simulink model "ControlOptimoInverso"  (R2025a)
settings: Solver=ode8  StartTime=0.0  StopTime=100  FixedStep=1e-3  RelTol=1e-3
libraries: simulink x1, spsRMSLib x1
settings Model: Creator=440G5  LastModifiedBy=440G5

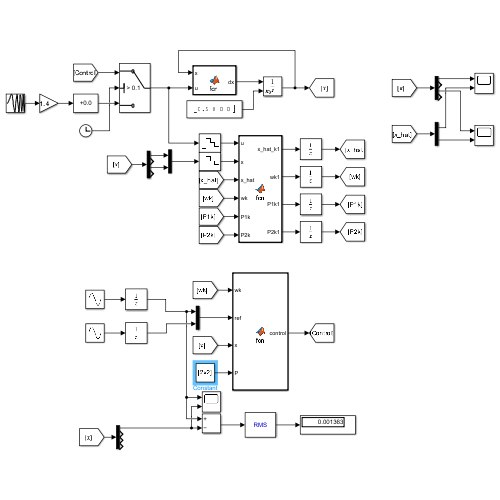
[thumbnail: Simulink's stored preview of the top-level diagram]
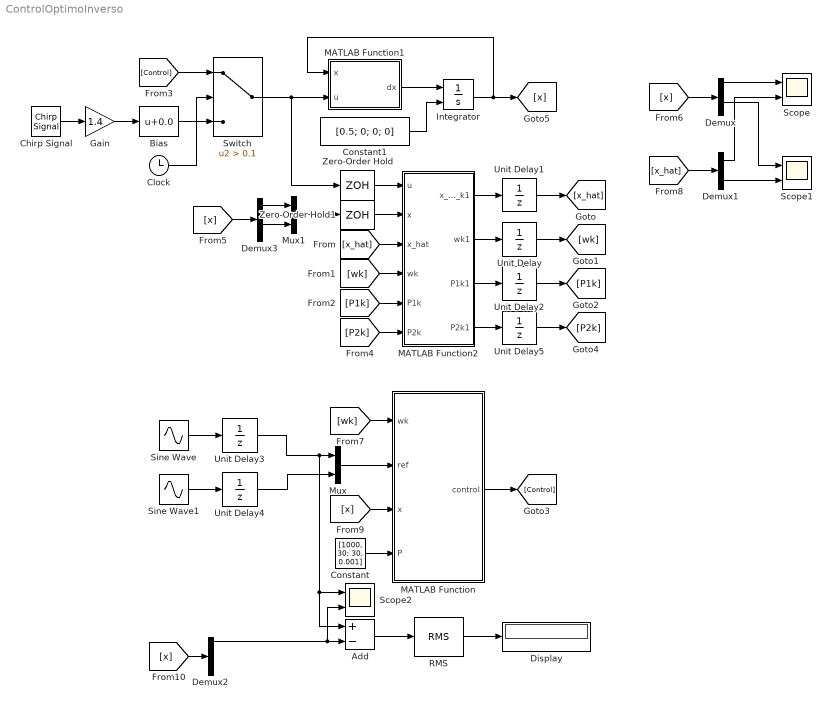
== system ControlOptimoInverso ==
  Add : Sum  Inputs=+-
  Bias : Bias  Bias=0.0  SaturateOnIntegerOverflow=off
  Chirp Signal : simulink/Sources/Chirp Signal  f1=0.08  T=10  f2=1
  Clock : Clock
      settings: Decimation=5
  Constant : Constant  Value=[1000, 30; 30, 0.001]
  Constant1 : Constant  Value=[0.5; 0; 0; 0]
  Demux : Demux
  Demux1 : Demux  Outputs=2
  Demux2 : Demux
  Demux3 : Demux
  Display : Display
  Gain : Gain  Gain=1.4
  Integrator : Integrator  InitialConditionSource=external
  MATLAB Function : MATLAB Function  TreatAsAtomicUnit=on
  MATLAB Function1 : MATLAB Function  TreatAsAtomicUnit=on
  MATLAB Function2 : MATLAB Function  TreatAsAtomicUnit=on
  Mux : Mux  Inputs=2
  Mux1 : Mux  Inputs=2
  RMS : spsRMSLib/RMS  TrueRMS=on  Freq=60  RMSInit=120  Ts=0
  Scope : Scope  NumInputPorts=2
      settings: ActiveDisplayYMinimum=-0.41183517995151714  ActiveDisplayYMaximum=0.922457634321867
  Scope1 : Scope  NumInputPorts=2
      settings: ActiveDisplayYMinimum=-0.72359460835221556  ActiveDisplayYMaximum=1.2933274161774539
  Scope2 : Scope  NumInputPorts=2
      settings: ActiveDisplayYMinimum=-0.92610552404399937  ActiveDisplayYMaximum=0.97588104782378549  DataLoggingVariableName=ScopeData2
  Sine Wave : Sin  Amplitude=0.35  SampleTime=0
  Sine Wave1 : Sin  Amplitude=0.5  SampleTime=0
  Switch : Switch  Criteria=u2 > Threshold  Threshold=0.1  SaturateOnIntegerOverflow=off  InputSameDT=off
  Unit Delay : UnitDelay  InitialCondition=[rand(1,4)]  SampleTime=-1  HasFrameUpgradeWarning=on
  Unit Delay1 : UnitDelay  SampleTime=-1  HasFrameUpgradeWarning=on
  Unit Delay2 : UnitDelay  InitialCondition=eye(2)*5e4  SampleTime=-1  HasFrameUpgradeWarning=on
  Unit Delay3 : UnitDelay  SampleTime=-1  HasFrameUpgradeWarning=on
  Unit Delay4 : UnitDelay  SampleTime=-1  HasFrameUpgradeWarning=on
  Unit Delay5 : UnitDelay  InitialCondition=eye(2)*5e4  SampleTime=-1  HasFrameUpgradeWarning=on
  Zero-Order Hold : ZeroOrderHold  SampleTime=-1
  Zero-Order Hold1 : ZeroOrderHold  SampleTime=-1
  wires:
  Chirp Signal/1 -> Gain/1
  Gain/1 -> Bias/1
  Bias/1 -> Switch/3
  Clock/1 -> Switch/2
  [Control] -> Switch/1
  MATLAB Function/1(control) -> [Control]
  Mux/1 -> MATLAB Function/2(ref)
  Constant/1 -> MATLAB Function/4(P)
  Sine Wave/1 -> Unit Delay3/1
  Sine Wave1/1 -> Unit Delay4/1
  Unit Delay3/1 -> Add/1, Scope2/1, Mux/1
  Unit Delay4/1 -> Mux/2
  [wk] -> MATLAB Function/1(wk)
  Unit Delay1/1 -> [x_hat]
  MATLAB Function2/2(wk1) -> Unit Delay/1
  [x] -> Demux/1
  [P2k] -> MATLAB Function2/6(P2k)
  Demux1/1 -> Scope/2
  [x_hat] -> Demux1/1
  MATLAB Function2/3(P1k1) -> Unit Delay2/1
  [wk] -> MATLAB Function2/4(wk)
  Unit Delay5/1 -> [P2k]
  Constant1/1 -> Integrator/2
  Demux1/2 -> Scope1/2
  Integrator/1 -> [x], MATLAB Function1/1(x)
  MATLAB Function2/1(x_hat_k1) -> Unit Delay1/1
  MATLAB Function1/1(dx) -> Integrator/1
  Zero-Order Hold/1 -> MATLAB Function2/1(u)
  Unit Delay/1 -> [wk]
  Unit Delay2/1 -> [P1k]
  [x_hat] -> MATLAB Function2/3(x_hat)
  Demux/1 -> Scope/1
  MATLAB Function2/4(P2k1) -> Unit Delay5/1
  Zero-Order Hold1/1 -> MATLAB Function2/2(x)
  [P1k] -> MATLAB Function2/5(P1k)
  [x] -> MATLAB Function/3(x)
  [x] -> Demux2/1
  Switch/1 -> Zero-Order Hold/1, MATLAB Function1/2(u)
  Demux3/1 -> Mux1/1
  Mux1/1 -> Zero-Order Hold1/1
  [x] -> Demux3/1
  Demux3/3 -> Mux1/2
  Demux/3 -> Scope1/1
  Demux2/1 -> Scope2/2, Add/2
  Add/1 -> RMS/1
  RMS/1 -> Display/1

== matlab function ControlOptimoInverso/MATLAB Function1 ==
  data: x input; u input; dx output
function dx = fcn(x, u)

m1 = 1;
m2 = 2;
k1 = 2;
k2 = 3;
b1 = 0.2;
b2 = 0.4;

dx1 = x(3);
dx2 = x(4);
dx3 = u/m1 -(k1/m1)*x(1) + (k1/m1)*x(2) -(b1/m1)*x(3) + (b1/m1)*x(4);
dx4 = (k1/m2)*x(1) - (k1/m2)*x(2) + (b1/m2)*x(3) -(b1/m2)*x(4) -(k2/m2)*x(2) -(b2/m2)*x(4);

dx = [dx1; dx2; dx3; dx4];

% function dx  = fcn(x, u)
% g = 9.81;  
% l = 1;     
% m = 1;     
% b = 0.5;   
% 
% x1 = x(1);  
% x2 = x(2);
% 
% dx1 = x2;
% dx2 = (g/l)*sin(x1) - (b/(m*l^2))*x2 + u/(m*l^2);
% 
% dx = [dx1; dx2];
% 
% y = x1;

== matlab function ControlOptimoInverso/MATLAB Function ==
  data: wk input; control output; ref input; x input; P input
function control  = fcn(wk, ref, x, P)

%% Constant weights
w_1 = 0.15;

%% Neural model
f1 = [wk(1)*tanh(x(2)) + wk(2)*tanh(x(1)); wk(3)*tanh(x(1)) + wk(4)*tanh(x(2))];
g1 = [0; w_1];

%% Control law
R = 1;
control = -1/2*(R+1/2*g1'*P*g1)\g1'*P*(f1 -[ref(1); ref(2)]);
end

== matlab function ControlOptimoInverso/MATLAB Function2 ==
  data: u input; x input; x_hat input; wk input; P1k input; P2k input; x_hat_k1 output; wk1 output; P1k1 output; P2k1 output
function [x_hat_k1, wk1, P1k1, P2k1] = fcn(u, x, x_hat, wk, P1k, P2k)

%% Constants weights
w_1 = 0.15;

%% Neural states
x_hat_k_1 = wk(1)*tanh(x(2)) + wk(2)*tanh(x(1));
x_hat_k_2 = wk(3)*tanh(x(1)) + wk(4)*tanh(x(2)) + w_1*u;
x_hat_k1 = [x_hat_k_1; x_hat_k_2];

%% H matrix coefficients
H1 = [tanh(x(2)) tanh(x(1))]';
H2 = [tanh(x(1)) tanh(x(2))]';

%% EKF computation per each state
Q1 = eye(2)*5e3;
R1 = 6e3;

Q2 = eye(2)*5e3;
R2 = 6e3;

% error
error = x - x_hat;

% First Filter
K1 = P1k*H1/(R1 + H1'*P1k*H1);
w1k1 = [wk(1); wk(2)] + K1*error(1);
P1k1 = P1k - K1*H1'*P1k + Q1;

% Second Filter
K2 = P2k*H2/(R2 + H2'*P2k*H2);
w2k1 = [wk(3); wk(4)] + K2*error(2);
P2k1 = P2k - K2*H2'*P2k + Q2;

wk1 = [w1k1; w2k1];
